simulink model "Three_Tank_System_Simulation_V1"  (R2019a)
settings: Solver=VariableStepAuto  StartTime=0.0  StopTime=10.0  RelTol=1e-3
values from neighbouring files (symbols this model uses):
  E_Valve_State_CISO : value not decoded    [Three_Tank_V1.sldd]
  E_Valve_State_COSI : value not decoded    [Three_Tank_V1.sldd]
libraries: simulink x15
settings Model: DataDictionary=Three_Tank_V1.sldd  Creator=rdkluijv  LastModifiedBy=rdkluijv

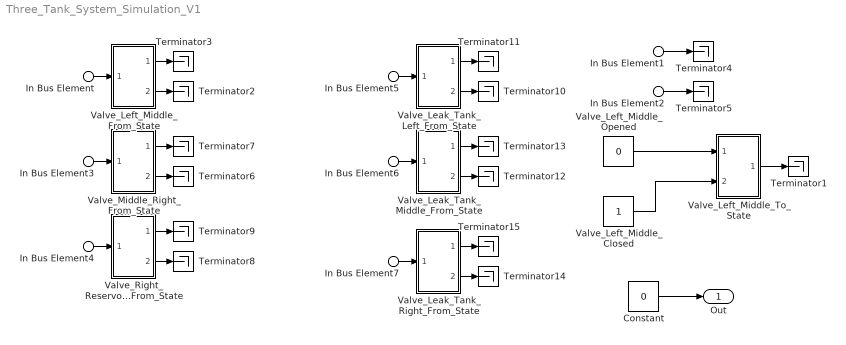
== system Three_Tank_System_Simulation_V1 ==
  In Bus Element1 : Inport  PortName=In  Element=Pump_Tank_Left
  In Bus Element2 : Inport  PortName=In  Element=Pump_Tank_Right
  In Bus Element : Inport  PortName=In  Element=Valve_Tank_Left_Middle.State
  In Bus Element3 : Inport  PortName=In  Element=Valve_Tank_Middle_Right.State
  In Bus Element4 : Inport  PortName=In  Element=Valve_Tank_Right_Reservoir.State
  In Bus Element5 : Inport  PortName=In  Element=Valve_Leak_Tank_Left.State
  In Bus Element6 : Inport  PortName=In  Element=Valve_Leak_Tank_Right.State
  In Bus Element7 : Inport  PortName=In  Element=Valve_Leak_Tank_Middle.State
  Constant : Constant  Value=0  OutDataTypeStr=Bus: Bus_CISO
  Terminator{1..15} (15 alike) : Terminator
  Valve_Leak_Tank_Left_From_State : Subsystem
  Valve_Leak_Tank_Middle_From_State : Subsystem
  Valve_Leak_Tank_Right_From_State : Subsystem
  Valve_Left_Middle_Closed : Constant  OutDataTypeStr=boolean
  Valve_Left_Middle_From_State : Subsystem
  Valve_Left_Middle_Opened : Constant  Value=0  OutDataTypeStr=boolean
  Valve_Left_Middle_To_State : Subsystem
  Valve_Middle_Right_From_State : Subsystem
  Valve_Right_Reservoir_From_State : Subsystem
  Out : Outport  OutDataTypeStr=Bus: Bus_CISO
  wires:
  Constant/1 -> Out/1
  Valve_Left_Middle_To_State/1(State) -> Terminator1/1
  Valve_Left_Middle_Opened/1 -> Valve_Left_Middle_To_State/1(Opened)
  Valve_Left_Middle_Closed/1 -> Valve_Left_Middle_To_State/2(Closed)
  In Bus Element/1 -> Valve_Left_Middle_From_State/1(State)
  Valve_Left_Middle_From_State/1(Close) -> Terminator3/1
  Valve_Left_Middle_From_State/2(Open) -> Terminator2/1
  In Bus Element2/1 -> Terminator5/1
  In Bus Element1/1 -> Terminator4/1
  Valve_Middle_Right_From_State/2(Open) -> Terminator6/1
  Valve_Middle_Right_From_State/1(Close) -> Terminator7/1
  In Bus Element3/1 -> Valve_Middle_Right_From_State/1(State)
  Valve_Right_Reservoir_From_State/1(Close) -> Terminator9/1
  Valve_Right_Reservoir_From_State/2(Open) -> Terminator8/1
  Valve_Leak_Tank_Left_From_State/2(Open) -> Terminator10/1
  Valve_Leak_Tank_Left_From_State/1(Close) -> Terminator11/1
  Valve_Leak_Tank_Middle_From_State/1(Close) -> Terminator13/1
  Valve_Leak_Tank_Middle_From_State/2(Open) -> Terminator12/1
  Valve_Leak_Tank_Right_From_State/2(Open) -> Terminator14/1
  Valve_Leak_Tank_Right_From_State/1(Close) -> Terminator15/1
  In Bus Element4/1 -> Valve_Right_Reservoir_From_State/1(State)
  In Bus Element5/1 -> Valve_Leak_Tank_Left_From_State/1(State)
  In Bus Element6/1 -> Valve_Leak_Tank_Middle_From_State/1(State)
  In Bus Element7/1 -> Valve_Leak_Tank_Right_From_State/1(State)

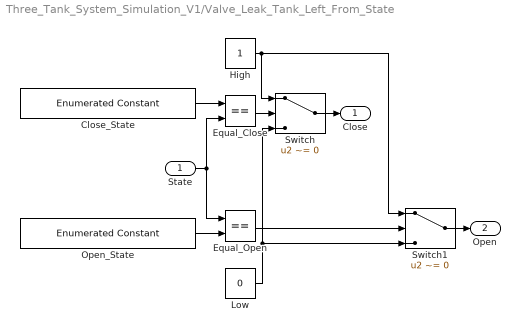
== system Three_Tank_System_Simulation_V1/Valve_Leak_Tank_Left_From_State ==
  State : Inport
  Close_State : simulink/Sources/Enumerated Constant  OutDataTypeStr=Enum: E_Valve_State_COSI  Value=E_Valve_State_COSI.Close  SampleTime=inf
      settings: SourceProductName=Simulink
  Equal_Close : RelationalOperator  Operator===  OutDataTypeStr=boolean  RndMeth=Simplest
  Equal_Open : RelationalOperator  Operator===  OutDataTypeStr=boolean  RndMeth=Simplest
  High : Constant  OutDataTypeStr=boolean
  Low : Constant  Value=0  OutDataTypeStr=boolean
  Open_State : simulink/Sources/Enumerated Constant  OutDataTypeStr=Enum: E_Valve_State_COSI  Value=E_Valve_State_COSI.Open  SampleTime=inf
      settings: SourceProductName=Simulink
  Switch : Switch  Criteria=u2 ~= 0  OutDataTypeStr=boolean
  Switch1 : Switch  Criteria=u2 ~= 0  OutDataTypeStr=boolean
  Close : Outport
  Open : Outport  Port=2
  wires:
  Close_State/1 -> Equal_Close/1
  Equal_Close/1 -> Switch/2
  Switch1/1 -> Open/1
  Equal_Open/1 -> Switch1/2
  Open_State/1 -> Equal_Open/2
  High/1 -> Switch/1, Switch1/1
  State/1 -> Equal_Open/1, Equal_Close/2
  Switch/1 -> Close/1
  Low/1 -> Switch1/3, Switch/3

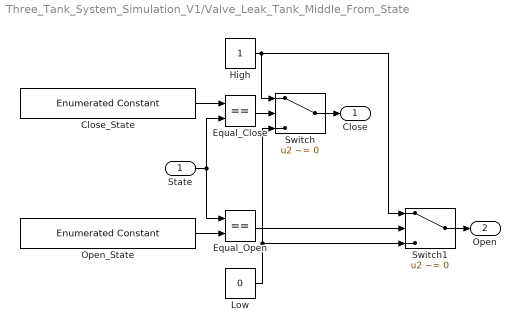
== system Three_Tank_System_Simulation_V1/Valve_Leak_Tank_Middle_From_State ==
  State : Inport
  Close_State : simulink/Sources/Enumerated Constant  OutDataTypeStr=Enum: E_Valve_State_COSI  Value=E_Valve_State_COSI.Close  SampleTime=inf
      settings: SourceProductName=Simulink
  Equal_Close : RelationalOperator  Operator===  OutDataTypeStr=boolean  RndMeth=Simplest
  Equal_Open : RelationalOperator  Operator===  OutDataTypeStr=boolean  RndMeth=Simplest
  High : Constant  OutDataTypeStr=boolean
  Low : Constant  Value=0  OutDataTypeStr=boolean
  Open_State : simulink/Sources/Enumerated Constant  OutDataTypeStr=Enum: E_Valve_State_COSI  Value=E_Valve_State_COSI.Open  SampleTime=inf
      settings: SourceProductName=Simulink
  Switch : Switch  Criteria=u2 ~= 0  OutDataTypeStr=boolean
  Switch1 : Switch  Criteria=u2 ~= 0  OutDataTypeStr=boolean
  Close : Outport
  Open : Outport  Port=2
  wires:
  Low/1 -> Switch/3, Switch1/3
  Switch/1 -> Close/1
  State/1 -> Equal_Close/2, Equal_Open/1
  High/1 -> Switch1/1, Switch/1
  Open_State/1 -> Equal_Open/2
  Equal_Open/1 -> Switch1/2
  Switch1/1 -> Open/1
  Equal_Close/1 -> Switch/2
  Close_State/1 -> Equal_Close/1

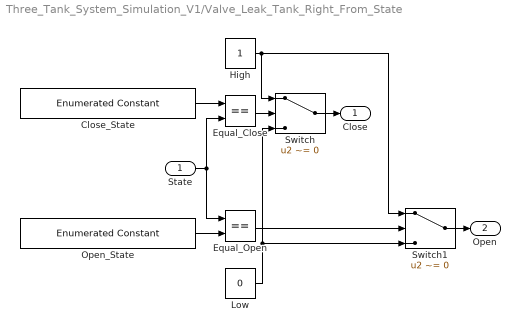
== system Three_Tank_System_Simulation_V1/Valve_Leak_Tank_Right_From_State ==
  State : Inport
  Close_State : simulink/Sources/Enumerated Constant  OutDataTypeStr=Enum: E_Valve_State_COSI  Value=E_Valve_State_COSI.Close  SampleTime=inf
      settings: SourceProductName=Simulink
  Equal_Close : RelationalOperator  Operator===  OutDataTypeStr=boolean  RndMeth=Simplest
  Equal_Open : RelationalOperator  Operator===  OutDataTypeStr=boolean  RndMeth=Simplest
  High : Constant  OutDataTypeStr=boolean
  Low : Constant  Value=0  OutDataTypeStr=boolean
  Open_State : simulink/Sources/Enumerated Constant  OutDataTypeStr=Enum: E_Valve_State_COSI  Value=E_Valve_State_COSI.Open  SampleTime=inf
      settings: SourceProductName=Simulink
  Switch : Switch  Criteria=u2 ~= 0  OutDataTypeStr=boolean
  Switch1 : Switch  Criteria=u2 ~= 0  OutDataTypeStr=boolean
  Close : Outport
  Open : Outport  Port=2
  wires:
  Close_State/1 -> Equal_Close/1
  Equal_Close/1 -> Switch/2
  Switch1/1 -> Open/1
  Equal_Open/1 -> Switch1/2
  Open_State/1 -> Equal_Open/2
  High/1 -> Switch/1, Switch1/1
  State/1 -> Equal_Open/1, Equal_Close/2
  Switch/1 -> Close/1
  Low/1 -> Switch1/3, Switch/3

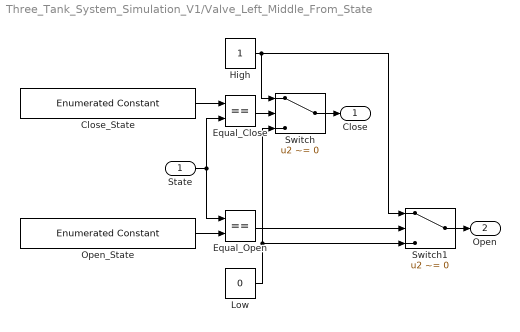
== system Three_Tank_System_Simulation_V1/Valve_Left_Middle_From_State ==
  State : Inport
  Close_State : simulink/Sources/Enumerated Constant  OutDataTypeStr=Enum: E_Valve_State_COSI  Value=E_Valve_State_COSI.Close  SampleTime=inf
      settings: SourceProductName=Simulink
  Equal_Close : RelationalOperator  Operator===  OutDataTypeStr=boolean  RndMeth=Simplest
  Equal_Open : RelationalOperator  Operator===  OutDataTypeStr=boolean  RndMeth=Simplest
  High : Constant  OutDataTypeStr=boolean
  Low : Constant  Value=0  OutDataTypeStr=boolean
  Open_State : simulink/Sources/Enumerated Constant  OutDataTypeStr=Enum: E_Valve_State_COSI  Value=E_Valve_State_COSI.Open  SampleTime=inf
      settings: SourceProductName=Simulink
  Switch : Switch  Criteria=u2 ~= 0  OutDataTypeStr=boolean
  Switch1 : Switch  Criteria=u2 ~= 0  OutDataTypeStr=boolean
  Close : Outport
  Open : Outport  Port=2
  wires:
  Low/1 -> Switch/3, Switch1/3
  Switch/1 -> Close/1
  State/1 -> Equal_Close/2, Equal_Open/1
  High/1 -> Switch1/1, Switch/1
  Open_State/1 -> Equal_Open/2
  Equal_Open/1 -> Switch1/2
  Switch1/1 -> Open/1
  Equal_Close/1 -> Switch/2
  Close_State/1 -> Equal_Close/1

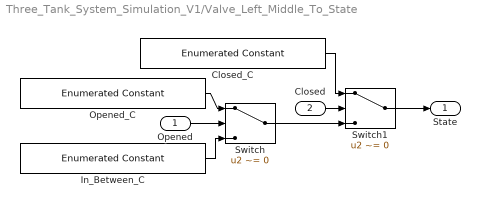
== system Three_Tank_System_Simulation_V1/Valve_Left_Middle_To_State ==
  Opened : Inport  OutDataTypeStr=boolean
  Closed : Inport  Port=2
  Closed_C : simulink/Sources/Enumerated Constant  OutDataTypeStr=Enum: E_Valve_State_CISO  Value=E_Valve_State_CISO.Closed  SampleTime=inf
      settings: SourceProductName=Simulink
  In_Between_C : simulink/Sources/Enumerated Constant  OutDataTypeStr=Enum: E_Valve_State_CISO  Value=E_Valve_State_CISO.In_Between  SampleTime=inf
      settings: SourceProductName=Simulink
  Opened_C : simulink/Sources/Enumerated Constant  OutDataTypeStr=Enum: E_Valve_State_CISO  Value=E_Valve_State_CISO.Opened  SampleTime=inf
      settings: SourceProductName=Simulink
  Switch : Switch  Criteria=u2 ~= 0  OutDataTypeStr=Enum: E_Valve_State_CISO  InputSameDT=on
      settings: LockScale=on
  Switch1 : Switch  Criteria=u2 ~= 0  OutDataTypeStr=Enum: E_Valve_State_CISO  InputSameDT=on
  State : Outport
  wires:
  In_Between_C/1 -> Switch/3
  Opened_C/1 -> Switch/1
  Closed_C/1 -> Switch1/1
  Opened/1 -> Switch/2
  Switch/1 -> Switch1/3
  Switch1/1 -> State/1
  Closed/1 -> Switch1/2

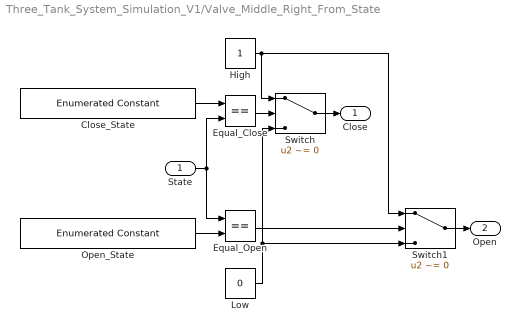
== system Three_Tank_System_Simulation_V1/Valve_Middle_Right_From_State ==
  State : Inport
  Close_State : simulink/Sources/Enumerated Constant  OutDataTypeStr=Enum: E_Valve_State_COSI  Value=E_Valve_State_COSI.Close  SampleTime=inf
      settings: SourceProductName=Simulink
  Equal_Close : RelationalOperator  Operator===  OutDataTypeStr=boolean  RndMeth=Simplest
  Equal_Open : RelationalOperator  Operator===  OutDataTypeStr=boolean  RndMeth=Simplest
  High : Constant  OutDataTypeStr=boolean
  Low : Constant  Value=0  OutDataTypeStr=boolean
  Open_State : simulink/Sources/Enumerated Constant  OutDataTypeStr=Enum: E_Valve_State_COSI  Value=E_Valve_State_COSI.Open  SampleTime=inf
      settings: SourceProductName=Simulink
  Switch : Switch  Criteria=u2 ~= 0  OutDataTypeStr=boolean
  Switch1 : Switch  Criteria=u2 ~= 0  OutDataTypeStr=boolean
  Close : Outport
  Open : Outport  Port=2
  wires:
  Close_State/1 -> Equal_Close/1
  Equal_Close/1 -> Switch/2
  Switch1/1 -> Open/1
  Equal_Open/1 -> Switch1/2
  Open_State/1 -> Equal_Open/2
  High/1 -> Switch/1, Switch1/1
  State/1 -> Equal_Open/1, Equal_Close/2
  Switch/1 -> Close/1
  Low/1 -> Switch1/3, Switch/3

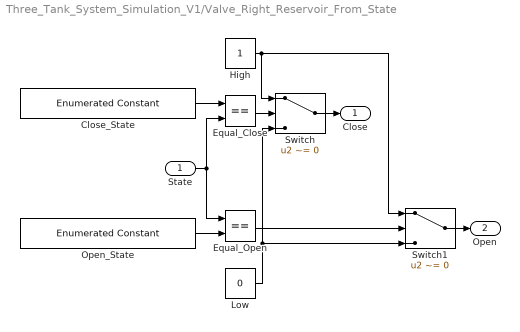
== system Three_Tank_System_Simulation_V1/Valve_Right_Reservoir_From_State ==
  State : Inport
  Close_State : simulink/Sources/Enumerated Constant  OutDataTypeStr=Enum: E_Valve_State_COSI  Value=E_Valve_State_COSI.Close  SampleTime=inf
      settings: SourceProductName=Simulink
  Equal_Close : RelationalOperator  Operator===  OutDataTypeStr=boolean  RndMeth=Simplest
  Equal_Open : RelationalOperator  Operator===  OutDataTypeStr=boolean  RndMeth=Simplest
  High : Constant  OutDataTypeStr=boolean
  Low : Constant  Value=0  OutDataTypeStr=boolean
  Open_State : simulink/Sources/Enumerated Constant  OutDataTypeStr=Enum: E_Valve_State_COSI  Value=E_Valve_State_COSI.Open  SampleTime=inf
      settings: SourceProductName=Simulink
  Switch : Switch  Criteria=u2 ~= 0  OutDataTypeStr=boolean
  Switch1 : Switch  Criteria=u2 ~= 0  OutDataTypeStr=boolean
  Close : Outport
  Open : Outport  Port=2
  wires:
  Low/1 -> Switch/3, Switch1/3
  Switch/1 -> Close/1
  State/1 -> Equal_Close/2, Equal_Open/1
  High/1 -> Switch1/1, Switch/1
  Open_State/1 -> Equal_Open/2
  Equal_Open/1 -> Switch1/2
  Switch1/1 -> Open/1
  Equal_Close/1 -> Switch/2
  Close_State/1 -> Equal_Close/1
